simulink subsystem "Flow_meter_L_s"  (R2022a)
settings: Solver=VariableStepAuto  StartTime=0.0  StopTime=10.0  RelTol=1e-3
libraries: fl_lib x2, nesl_utility x1
settings Model: Creator=simmo536  LastModifiedBy=simmo536

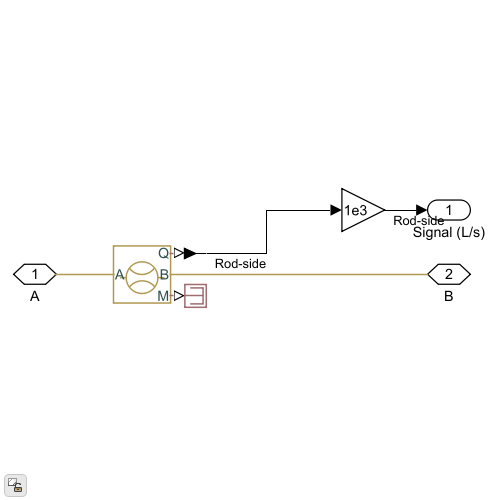
[thumbnail: Simulink's stored preview of the top-level diagram]
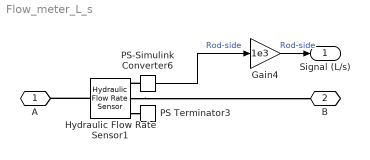
== system Flow_meter_L_s ==
  Gain4 : Gain  Gain=1e3
  Hydraulic Flow Rate Sensor1 : fl_lib/Hydraulic/Hydraulic Sensors/Hydraulic Flow Rate Sensor
      settings: SourceProductBaseCode=PW,SS,VE
  PS Terminator3 : fl_lib/Physical Signals/Sinks/PS Terminator
      settings: SourceProductBaseCode=PW,SS,VE
  PS-Simulink Converter6 : nesl_utility/PS-Simulink Converter  PhysicalDomain=network_engine_domain  SubClassName=ps_output  LeftPortType=input  RightPortType=output  PseudoPeriodic=off  Frequencies=[]  VectorFormat=1-D array  Unit=inherit  AffineConversion=off
      settings: SourceProductBaseCode=SS,PW,VE
  A : PMIOPort  Side=Left
  B : PMIOPort  Port=2  Side=Right
  Signal (L/s) : Outport
  wires:
  Gain4/1 -> Signal (L/s)/1  "Rod-side"
  PS-Simulink Converter6/1 -> Gain4/1  "Rod-side"
  connections:
  PS-Simulink Converter6/LConn1 -- Hydraulic Flow Rate Sensor1/RConn1
  Hydraulic Flow Rate Sensor1/RConn3 -- PS Terminator3/LConn1
  Hydraulic Flow Rate Sensor1/LConn1 -- A/RConn1
  Hydraulic Flow Rate Sensor1/RConn2 -- B/RConn1
